simulink model "SiMoDronesBebopRos_student"  (R2021a)
settings: Solver=FixedStepAuto  StartTime=0  StopTime=35  FixedStep=0.005  MaxStep=1e-3  MinStep=5e-5  RelTol=1e-5  AbsTol=1e-5
StopFcn:
  | %data_bebop;
  | save_and_plot_data
values from neighbouring files (symbols this model uses):
  aero =     [test1_p1.mat]    (also in test2_P2.mat; test3_pd.mat; test4_lat.mat; xtest4_lat.mat)
  controlGains =     [test1_p1.mat]    (also in test2_P2.mat; test3_pd.mat; test4_lat.mat; xtest4_lat.mat)
  drone =     [test1_p1.mat]    (also in test2_P2.mat; test3_pd.mat; test4_lat.mat; xtest4_lat.mat)
  init_state =     [test1_p1.mat]    (also in test2_P2.mat; test3_pd.mat; test4_lat.mat; xtest4_lat.mat)
  K = place(A,B,P0)    [Control.m]    (also in test1_p1.mat = [0.637104994903 0.356778797146]; test2_P2.mat = [0.637104994903 0.356778797146]; test3_pd.mat = [0.637104994903 0.356778797146]; test4_lat.mat = [0.637104994903 0.356778797146])
  Kd = 3.806    [Control.m]    (also in test1_p1.mat = 5.726; test2_P2.mat = 5.726; test3_pd.mat = 5.726; test4_lat.mat = 5.726)
  Kdd = 2*sg*om*tau-1    (= 0.98)    [Control.m]    (also in test1_p1.mat = 1.509; test2_P2.mat = 1.509; test3_pd.mat; test4_lat.mat = 1.509)
  Ki = 37.39    [Control.m]    (also in test1_p1.mat = 83.71; test2_P2.mat = 83.71; test3_pd.mat = 83.71; test4_lat.mat = 83.71)
  Kp = 25.23    [Control.m]    (also in test1_p1.mat = 43.79; test2_P2.mat = 43.79; test3_pd.mat = 43.79; test4_lat.mat = 43.79)
  Kp1 = 4    [Control.m]    (also in test1_p1.mat; test2_P2.mat; test3_pd.mat; test4_lat.mat)
  Kp2 = 5.2071    [Control.m]    (also in test1_p1.mat; test2_P2.mat; test3_pd.mat; test4_lat.mat)
  Kpd = tau*om^2    (= 6.0612244898)    [Control.m]    (also in test1_p1.mat = 12.82; test2_P2.mat = 12.82; test3_pd.mat; test4_lat.mat = 12.82)
  measure =     [test1_p1.mat]    (also in test2_P2.mat; test3_pd.mat; test4_lat.mat; xtest4_lat.mat)
  motor =     [test1_p1.mat]    (also in test2_P2.mat; test3_pd.mat; test4_lat.mat; xtest4_lat.mat)
  N = K1    [Control.m]    (also in test1_p1.mat = 0.637104994903; test2_P2.mat = 0.637104994903; test3_pd.mat = 0.637104994903; test4_lat.mat = 0.637104994903)
  tau = 0.33    [Control.m]    (also in test1_p1.mat; test2_P2.mat; test3_pd.mat; test4_lat.mat)
  Te = Ts_optitrack    (= 0.02)    [Startup_bebop_ros.m]    (also in test1_p1.mat; test2_P2.mat; test3_pd.mat; test4_lat.mat)
  Te_topics_empty = 0.1    [Startup_bebop_ros.m]    (also in test1_p1.mat; test2_P2.mat; test3_pd.mat; test4_lat.mat)
  Ts_bebop = 5e-3    (= 0.005)    [Startup_bebop_ros.m]    (also in test1_p1.mat; test2_P2.mat; test3_pd.mat; test4_lat.mat)
  Ts_bebop_feedback = 2e-1    (= 0.2)    [Startup_bebop_ros.m]    (also in test1_p1.mat; test2_P2.mat; test3_pd.mat; test4_lat.mat)
  Ts_optitrack = 2e-2    (= 0.02)    [Startup_bebop_ros.m]    (also in test1_p1.mat; test2_P2.mat; test3_pd.mat; test4_lat.mat)
undefined symbols (not defined in the file or in its folder): Angular, DiscIntNeverNeededParam, gcbh, Linear, sigbuilder_block, sldros_modeswitch
libraries: robotlib x15, simulink x9, pid_lib x8, vrlib x5, lib_isae_drones x4, aerolibanimutils x2, sharedtransform x2, aerolibobsolete x1, drones x1
(part 2 of 3)

== system SiMoDronesBebopRos_student/BEBOP/Model/Model/Bus Mapping1 ==
  Position : Inport
  Velocity : Inport  Port=2
  Attitude : Inport  Port=3
  Omega : Inport  Port=4
  Bus Creator : BusCreator  Inputs=12  OutDataTypeStr=Bus: BUS_bebop_pos_att
  Demux{,1..3} (4 alike) : Demux  Outputs=3
  pos_att_NED : Outport  OutDataTypeStr=Bus: BUS_bebop_pos_att  VectorParamsAs1DForOutWhenUnconnected=off
  wires:
  Position/1 -> Demux/1
  Demux/1 -> Bus Creator/1  "X"
  Demux/3 -> Bus Creator/3  "Z"
  Demux/2 -> Bus Creator/2  "Y"
  Velocity/1 -> Demux1/1
  Demux1/1 -> Bus Creator/4  "VX"
  Demux1/2 -> Bus Creator/5  "VY"
  Demux1/3 -> Bus Creator/6  "VZ"
  Attitude/1 -> Demux2/1
  Demux2/1 -> Bus Creator/7  "Phi"
  Demux2/2 -> Bus Creator/8  "Theta"
  Demux2/3 -> Bus Creator/9  "Psi"
  Omega/1 -> Demux3/1
  Demux3/1 -> Bus Creator/10  "p"
  Demux3/2 -> Bus Creator/11  "q"
  Demux3/3 -> Bus Creator/12  "r"
  Bus Creator/1 -> pos_att_NED/1

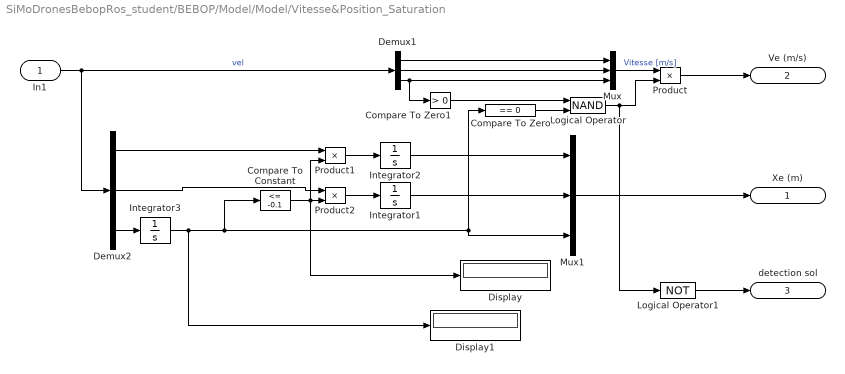
== system SiMoDronesBebopRos_student/BEBOP/Model/Model/Vitesse&Position_Saturation ==
  In1 : Inport
  Compare To Constant : simulink/Logic and Bit Operations/Compare To Constant  relop=<=  const=-0.1  OutDataTypeStr=boolean
  Compare To Zero : simulink/Logic and Bit Operations/Compare To Zero  relop===  OutDataTypeStr=boolean
  Compare To Zero1 : simulink/Logic and Bit Operations/Compare To Zero  relop=>  OutDataTypeStr=boolean
  Demux1 : Demux  Outputs=3
  Demux2 : Demux  Outputs=3
  Display : Display
  Display1 : Display
  Integrator1 : Integrator  InitialCondition=init_state.Pterre0(2)  UpperSaturationLimit=[Inf Inf 0]
  Integrator2 : Integrator  InitialCondition=init_state.Pterre0(1)  UpperSaturationLimit=[Inf Inf 0]
  Integrator3 : Integrator  InitialCondition=init_state.Pterre0(3)  LimitOutput=on  UpperSaturationLimit=[0]
  Logical Operator : Logic  Operator=NAND  AllPortsSameDT=off  OutDataTypeStr=boolean
  Logical Operator1 : Logic  Operator=NOT  AllPortsSameDT=off  OutDataTypeStr=boolean
  Mux : Mux  Inputs=3
  Mux1 : Mux  Inputs=3
  Product : Product  RndMeth=Zero
  Product1 : Product  RndMeth=Zero
  Product2 : Product  RndMeth=Zero
  Xe (m) : Outport  VectorParamsAs1DForOutWhenUnconnected=off
  Ve (m/s) : Outport  Port=2  VectorParamsAs1DForOutWhenUnconnected=off
  detection sol : Outport  Port=3  VectorParamsAs1DForOutWhenUnconnected=off
  wires:
  Compare To Zero1/1 -> Logical Operator/1
  Compare To Zero/1 -> Logical Operator/2
  Demux1/1 -> Mux/1
  Demux1/2 -> Mux/2
  Demux1/3 -> Mux/3, Compare To Zero1/1
  In1/1 -> Demux1/1, Demux2/1  "vel"
  Mux/1 -> Product/1  "Vitesse [m/s]"
  Product/1 -> Ve (m/s)/1
  Integrator1/1 -> Mux1/2
  Demux2/3 -> Integrator3/1
  Integrator3/1 -> Display1/1, Compare To Constant/1, Compare To Zero/1, Mux1/3
  Integrator2/1 -> Mux1/1
  Product1/1 -> Integrator2/1
  Demux2/1 -> Product1/1
  Product2/1 -> Integrator1/1
  Demux2/2 -> Product2/1
  Compare To Constant/1 -> Product1/2, Display/1, Product2/2
  Mux1/1 -> Xe (m)/1
  Logical Operator/1 -> Logical Operator1/1, Product/2
  Logical Operator1/1 -> detection sol/1

== system SiMoDronesBebopRos_student/Guidance & Control /Position Control/Control z/P controller - 1st order system ==
  note: Model
  note: Bebop simulation
  Zref : Inport
  Vz : Inport  Port=2
  Z : Inport  Port=3
  Integrator : Integrator  InitialCondition=-1.5
  PID Controller : pid_lib/PID Controller  Controller=P  Form=Parallel  TimeDomain=Discrete-time  UseExternalTs=off  SampleTime=0.02  IntegratorMethod=Forward Euler  FilterMethod=Forward Euler  ControllerParametersSource=internal  P=Kp1  I=1  D=0.9800  UseFilter=off  N=100  TunerSelectOption=Transfer Function Based (PID Tuner App)  InitialConditionSource=internal  InitialConditionForIntegrator=0  InitialConditionForFilter=0  DifferentiatorICPrevScaledInput=0  ExternalReset=none  TrackingMode=off  Kt=1  LimitOutput=off  SatLimitsSource=internal  UpperSaturationLimit=inf  LowerSaturationLimit=-inf  LinearizeAsGain=on  AntiWindupMode=none  Kb=1  POutMin=[]  POutMax=[]  IOutMin=[]  IOutMax=[]  DOutMin=[]  DOutMax=[]  NOutMin=[]  NOutMax=[]  SumOutMin=[]  SumOutMax=[]  SaturationOutMin=[]  SaturationOutMax=[]  PParamMin=[]  PParamMax=[]  IParamMin=[]  IParamMax=[]  DParamMin=[]  DParamMax=[]  NParamMin=[]  NParamMax=[]  KbParamMin=[]  KbParamMax=[]  KtParamMin=[]  KtParamMax=[]  KbOutMin=[]  KbOutMax=[]  KtOutMin=[]  KtOutMax=[]  IntegratorOutMin=[]  IntegratorOutMax=[]  FilterOutMin=[]  FilterOutMax=[]  SumI1OutMin=[]  SumI1OutMax=[]  SumI2OutMin=[]  SumI2OutMax=[]  SumI3OutMin=[]  SumI3OutMax=[]  SumI4OutMin=[]  SumI4OutMax=[]  SumDOutMin=[]  SumDOutMax=[]  DifferentiatorOutMin=[]  DifferentiatorOutMax=[]  FilterDiffOutCoefMin=[]  FilterDiffOutCoefMax=[]  ReciprocalOutMin=[]  ReciprocalOutMax=[]  SumDenOutMin=[]  SumDenOutMax=[]  SumNumOutMin=[]  SumNumOutMax=[]  DivideOutMin=[]  DivideOutMax=[]  UdiffTsProdOutMin=[]  UdiffTsProdOutMax=[]  NTsProdOutMin=[]  NTsProdOutMax=[]  UintegralTsProdOutMin=[]  UintegralTsProdOutMax=[]  UngainTsProdOutMin=[]  UngainTsProdOutMax=[]  IntegratorContinuousStateAttributes=''  IntegratorStateMustResolveToSignalObject=off  IntegratorRTWStateStorageClass=Auto  FilterContinuousStateAttributes=''  FilterStateMustResolveToSignalObject=off  FilterRTWStateStorageClass=Auto  ParallelPVariant=InternalParameters  IdealPVariant=Disabled  IVariant=Disabled  DVariant=Disabled  IntegratorVariant=Disabled  SatVariant=Disabled  AWVariant=Disabled  PCopyVariant=Disabled  TRVariant=Disabled  FdbkBlocksVariant=Forward  IdealPFdbkVariant=Disabled  SatFdbkVariant=Disabled  DerivativeFilterVariant=Disabled  NVariant=Disabled  NCopyVariant=Disabled_SignalSpec  FilterICVariant=Disabled  IntegratorICVariant=Disabled  ExternalResetVariant=Disabled  TRSumVariant=Passthrough  SumFdbkVariant=Disabled  SumVariant=Passthrough_P  TsampFilterVariant=InternalTs  TsampNgainVariant=Passthrough  TsampIntegralVariant=Disabled_SignalSpec  ExternalSaturationOutDataTypeStr=Inherit: Same as second input
  PID Controller1 : pid_lib/PID Controller  Controller=P  Form=Parallel  TimeDomain=Discrete-time  UseExternalTs=off  SampleTime=0.02  IntegratorMethod=Forward Euler  FilterMethod=Forward Euler  ControllerParametersSource=internal  P=Kp1  I=1  D=0.9800  UseFilter=off  N=100  TunerSelectOption=Transfer Function Based (PID Tuner App)  InitialConditionSource=internal  InitialConditionForIntegrator=0  InitialConditionForFilter=0  DifferentiatorICPrevScaledInput=0  ExternalReset=none  TrackingMode=off  Kt=1  LimitOutput=off  SatLimitsSource=internal  UpperSaturationLimit=inf  LowerSaturationLimit=-inf  LinearizeAsGain=on  AntiWindupMode=none  Kb=1  POutMin=[]  POutMax=[]  IOutMin=[]  IOutMax=[]  DOutMin=[]  DOutMax=[]  NOutMin=[]  NOutMax=[]  SumOutMin=[]  SumOutMax=[]  SaturationOutMin=[]  SaturationOutMax=[]  PParamMin=[]  PParamMax=[]  IParamMin=[]  IParamMax=[]  DParamMin=[]  DParamMax=[]  NParamMin=[]  NParamMax=[]  KbParamMin=[]  KbParamMax=[]  KtParamMin=[]  KtParamMax=[]  KbOutMin=[]  KbOutMax=[]  KtOutMin=[]  KtOutMax=[]  IntegratorOutMin=[]  IntegratorOutMax=[]  FilterOutMin=[]  FilterOutMax=[]  SumI1OutMin=[]  SumI1OutMax=[]  SumI2OutMin=[]  SumI2OutMax=[]  SumI3OutMin=[]  SumI3OutMax=[]  SumI4OutMin=[]  SumI4OutMax=[]  SumDOutMin=[]  SumDOutMax=[]  DifferentiatorOutMin=[]  DifferentiatorOutMax=[]  FilterDiffOutCoefMin=[]  FilterDiffOutCoefMax=[]  ReciprocalOutMin=[]  ReciprocalOutMax=[]  SumDenOutMin=[]  SumDenOutMax=[]  SumNumOutMin=[]  SumNumOutMax=[]  DivideOutMin=[]  DivideOutMax=[]  UdiffTsProdOutMin=[]  UdiffTsProdOutMax=[]  NTsProdOutMin=[]  NTsProdOutMax=[]  UintegralTsProdOutMin=[]  UintegralTsProdOutMax=[]  UngainTsProdOutMin=[]  UngainTsProdOutMax=[]  IntegratorContinuousStateAttributes=''  IntegratorStateMustResolveToSignalObject=off  IntegratorRTWStateStorageClass=Auto  FilterContinuousStateAttributes=''  FilterStateMustResolveToSignalObject=off  FilterRTWStateStorageClass=Auto  ParallelPVariant=InternalParameters  IdealPVariant=Disabled  IVariant=Disabled  DVariant=Disabled  IntegratorVariant=Disabled  SatVariant=Disabled  AWVariant=Disabled  PCopyVariant=Disabled  TRVariant=Disabled  FdbkBlocksVariant=Forward  IdealPFdbkVariant=Disabled  SatFdbkVariant=Disabled  DerivativeFilterVariant=Disabled  NVariant=Disabled  NCopyVariant=Disabled_SignalSpec  FilterICVariant=Disabled  IntegratorICVariant=Disabled  ExternalResetVariant=Disabled  TRSumVariant=Passthrough  SumFdbkVariant=Disabled  SumVariant=Passthrough_P  TsampFilterVariant=InternalTs  TsampNgainVariant=Passthrough  TsampIntegralVariant=Disabled_SignalSpec  ExternalSaturationOutDataTypeStr=Inherit: Same as second input
  Scope : Scope  NumInputPorts=2
  Scope1 : Scope  NumInputPorts=2
  Sum : Sum  Inputs=|+-
  Sum1 : Sum  Inputs=|+-
  To Workspace : ToWorkspace  VariableName=zmodel_P1  SaveFormat=Timeseries  SampleTime=0.02
  VZref : Outport  OutputWhenDisabled=reset  InitialOutput=0  VectorParamsAs1DForOutWhenUnconnected=off
  wires:
  Z/1 -> Sum/2, Scope/1  "zopti"
  PID Controller/1 -> VZref/1
  Sum/1 -> PID Controller/1
  Integrator/1 -> To Workspace/1, Scope/2, Sum1/2  "zmodel"
  PID Controller1/1 -> Scope1/2, Integrator/1  "Vzmodel"
  Vz/1 -> Scope1/1
  Sum1/1 -> PID Controller1/1
  Zref/1 -> Sum1/1, Sum/1

== system SiMoDronesBebopRos_student/Guidance & Control /Position Control/Control z/P controller - 2nd order system ==
  note: Model
  note: Bebop simulation
  Zref : Inport
  Vz : Inport  Port=2
  Z : Inport  Port=3
  Actuator dynamics : TransferFcn  Denominator=[tau 1]
  Integrator : Integrator  InitialCondition=-1.5
  PID Controller : pid_lib/PID Controller  Controller=P  Form=Parallel  TimeDomain=Discrete-time  UseExternalTs=off  SampleTime=0.02  IntegratorMethod=Forward Euler  FilterMethod=Forward Euler  ControllerParametersSource=internal  P=Kp2  I=1  D=1  UseFilter=on  N=100  TunerSelectOption=Transfer Function Based (PID Tuner App)  InitialConditionSource=internal  InitialConditionForIntegrator=0  InitialConditionForFilter=0  DifferentiatorICPrevScaledInput=0  ExternalReset=none  TrackingMode=off  Kt=1  LimitOutput=off  SatLimitsSource=internal  UpperSaturationLimit=inf  LowerSaturationLimit=-inf  LinearizeAsGain=on  AntiWindupMode=none  Kb=1  POutMin=[]  POutMax=[]  IOutMin=[]  IOutMax=[]  DOutMin=[]  DOutMax=[]  NOutMin=[]  NOutMax=[]  SumOutMin=[]  SumOutMax=[]  SaturationOutMin=[]  SaturationOutMax=[]  PParamMin=[]  PParamMax=[]  IParamMin=[]  IParamMax=[]  DParamMin=[]  DParamMax=[]  NParamMin=[]  NParamMax=[]  KbParamMin=[]  KbParamMax=[]  KtParamMin=[]  KtParamMax=[]  KbOutMin=[]  KbOutMax=[]  KtOutMin=[]  KtOutMax=[]  IntegratorOutMin=[]  IntegratorOutMax=[]  FilterOutMin=[]  FilterOutMax=[]  SumI1OutMin=[]  SumI1OutMax=[]  SumI2OutMin=[]  SumI2OutMax=[]  SumI3OutMin=[]  SumI3OutMax=[]  SumI4OutMin=[]  SumI4OutMax=[]  SumDOutMin=[]  SumDOutMax=[]  DifferentiatorOutMin=[]  DifferentiatorOutMax=[]  FilterDiffOutCoefMin=[]  FilterDiffOutCoefMax=[]  ReciprocalOutMin=[]  ReciprocalOutMax=[]  SumDenOutMin=[]  SumDenOutMax=[]  SumNumOutMin=[]  SumNumOutMax=[]  DivideOutMin=[]  DivideOutMax=[]  UdiffTsProdOutMin=[]  UdiffTsProdOutMax=[]  NTsProdOutMin=[]  NTsProdOutMax=[]  UintegralTsProdOutMin=[]  UintegralTsProdOutMax=[]  UngainTsProdOutMin=[]  UngainTsProdOutMax=[]  IntegratorContinuousStateAttributes=''  IntegratorStateMustResolveToSignalObject=off  IntegratorRTWStateStorageClass=Auto  FilterContinuousStateAttributes=''  FilterStateMustResolveToSignalObject=off  FilterRTWStateStorageClass=Auto  ParallelPVariant=InternalParameters  IdealPVariant=Disabled  IVariant=Disabled  DVariant=Disabled  IntegratorVariant=Disabled  SatVariant=Disabled  AWVariant=Disabled  PCopyVariant=Disabled  TRVariant=Disabled  FdbkBlocksVariant=Forward  IdealPFdbkVariant=Disabled  SatFdbkVariant=Disabled  DerivativeFilterVariant=Disabled  NVariant=Disabled  NCopyVariant=Disabled_SignalSpec  FilterICVariant=Disabled  IntegratorICVariant=Disabled  ExternalResetVariant=Disabled  TRSumVariant=Passthrough  SumFdbkVariant=Disabled  SumVariant=Passthrough_P  TsampFilterVariant=InternalTs  TsampNgainVariant=Passthrough  TsampIntegralVariant=Disabled_SignalSpec  ExternalSaturationOutDataTypeStr=Inherit: Same as second input
  PID Controller1 : pid_lib/PID Controller  Controller=P  Form=Parallel  TimeDomain=Discrete-time  UseExternalTs=off  SampleTime=0.02  IntegratorMethod=Forward Euler  FilterMethod=Forward Euler  ControllerParametersSource=internal  P=Kp2  I=1  D=1  UseFilter=on  N=100  TunerSelectOption=Transfer Function Based (PID Tuner App)  InitialConditionSource=internal  InitialConditionForIntegrator=0  InitialConditionForFilter=0  DifferentiatorICPrevScaledInput=0  ExternalReset=none  TrackingMode=off  Kt=1  LimitOutput=off  SatLimitsSource=internal  UpperSaturationLimit=inf  LowerSaturationLimit=-inf  LinearizeAsGain=on  AntiWindupMode=none  Kb=1  POutMin=[]  POutMax=[]  IOutMin=[]  IOutMax=[]  DOutMin=[]  DOutMax=[]  NOutMin=[]  NOutMax=[]  SumOutMin=[]  SumOutMax=[]  SaturationOutMin=[]  SaturationOutMax=[]  PParamMin=[]  PParamMax=[]  IParamMin=[]  IParamMax=[]  DParamMin=[]  DParamMax=[]  NParamMin=[]  NParamMax=[]  KbParamMin=[]  KbParamMax=[]  KtParamMin=[]  KtParamMax=[]  KbOutMin=[]  KbOutMax=[]  KtOutMin=[]  KtOutMax=[]  IntegratorOutMin=[]  IntegratorOutMax=[]  FilterOutMin=[]  FilterOutMax=[]  SumI1OutMin=[]  SumI1OutMax=[]  SumI2OutMin=[]  SumI2OutMax=[]  SumI3OutMin=[]  SumI3OutMax=[]  SumI4OutMin=[]  SumI4OutMax=[]  SumDOutMin=[]  SumDOutMax=[]  DifferentiatorOutMin=[]  DifferentiatorOutMax=[]  FilterDiffOutCoefMin=[]  FilterDiffOutCoefMax=[]  ReciprocalOutMin=[]  ReciprocalOutMax=[]  SumDenOutMin=[]  SumDenOutMax=[]  SumNumOutMin=[]  SumNumOutMax=[]  DivideOutMin=[]  DivideOutMax=[]  UdiffTsProdOutMin=[]  UdiffTsProdOutMax=[]  NTsProdOutMin=[]  NTsProdOutMax=[]  UintegralTsProdOutMin=[]  UintegralTsProdOutMax=[]  UngainTsProdOutMin=[]  UngainTsProdOutMax=[]  IntegratorContinuousStateAttributes=''  IntegratorStateMustResolveToSignalObject=off  IntegratorRTWStateStorageClass=Auto  FilterContinuousStateAttributes=''  FilterStateMustResolveToSignalObject=off  FilterRTWStateStorageClass=Auto  ParallelPVariant=InternalParameters  IdealPVariant=Disabled  IVariant=Disabled  DVariant=Disabled  IntegratorVariant=Disabled  SatVariant=Disabled  AWVariant=Disabled  PCopyVariant=Disabled  TRVariant=Disabled  FdbkBlocksVariant=Forward  IdealPFdbkVariant=Disabled  SatFdbkVariant=Disabled  DerivativeFilterVariant=Disabled  NVariant=Disabled  NCopyVariant=Disabled_SignalSpec  FilterICVariant=Disabled  IntegratorICVariant=Disabled  ExternalResetVariant=Disabled  TRSumVariant=Passthrough  SumFdbkVariant=Disabled  SumVariant=Passthrough_P  TsampFilterVariant=InternalTs  TsampNgainVariant=Passthrough  TsampIntegralVariant=Disabled_SignalSpec  ExternalSaturationOutDataTypeStr=Inherit: Same as second input
  Scope : Scope  NumInputPorts=2
  Scope1 : Scope  NumInputPorts=2
  Sum : Sum  Inputs=|+-
  Sum1 : Sum  Inputs=|+-
  To Workspace : ToWorkspace  VariableName=zmodel_P2  SaveFormat=Timeseries  SampleTime=0.02
  VZref : Outport  OutputWhenDisabled=reset  InitialOutput=0  VectorParamsAs1DForOutWhenUnconnected=off
  wires:
  Z/1 -> Sum/2, Scope/1  "zopti"
  Zref/1 -> Sum1/1, Sum/1
  PID Controller/1 -> VZref/1
  Sum/1 -> PID Controller/1
  Integrator/1 -> Sum1/2, To Workspace/1, Scope/2  "zmodel"
  Vz/1 -> Scope1/1
  Sum1/1 -> PID Controller1/1
  PID Controller1/1 -> Actuator dynamics/1  "Vzmodel"
  Actuator dynamics/1 -> Scope1/2, Integrator/1

== system SiMoDronesBebopRos_student/Guidance & Control /Position Control/Control z/PD controller - 2nd order system ==
  note: Model
  note: Bebop simulation
  Zref : Inport
  Vz : Inport  Port=2
  Z : Inport  Port=3
  Actuator dynamics : TransferFcn  Denominator=[tau 1]
  Integrator : Integrator  InitialCondition=-1.5
  PID Controller : pid_lib/PID Controller  Controller=PD  Form=Parallel  TimeDomain=Discrete-time  UseExternalTs=off  SampleTime=0.02  IntegratorMethod=Forward Euler  FilterMethod=Forward Euler  ControllerParametersSource=internal  P=Kpd  I=1  D=Kdd  UseFilter=off  N=100  TunerSelectOption=Transfer Function Based (PID Tuner App)  InitialConditionSource=internal  InitialConditionForIntegrator=0  InitialConditionForFilter=0  DifferentiatorICPrevScaledInput=0  ExternalReset=none  TrackingMode=off  Kt=1  LimitOutput=off  SatLimitsSource=internal  UpperSaturationLimit=inf  LowerSaturationLimit=-inf  LinearizeAsGain=on  AntiWindupMode=none  Kb=1  POutMin=[]  POutMax=[]  IOutMin=[]  IOutMax=[]  DOutMin=[]  DOutMax=[]  NOutMin=[]  NOutMax=[]  SumOutMin=[]  SumOutMax=[]  SaturationOutMin=[]  SaturationOutMax=[]  PParamMin=[]  PParamMax=[]  IParamMin=[]  IParamMax=[]  DParamMin=[]  DParamMax=[]  NParamMin=[]  NParamMax=[]  KbParamMin=[]  KbParamMax=[]  KtParamMin=[]  KtParamMax=[]  KbOutMin=[]  KbOutMax=[]  KtOutMin=[]  KtOutMax=[]  IntegratorOutMin=[]  IntegratorOutMax=[]  FilterOutMin=[]  FilterOutMax=[]  SumI1OutMin=[]  SumI1OutMax=[]  SumI2OutMin=[]  SumI2OutMax=[]  SumI3OutMin=[]  SumI3OutMax=[]  SumI4OutMin=[]  SumI4OutMax=[]  SumDOutMin=[]  SumDOutMax=[]  DifferentiatorOutMin=[]  DifferentiatorOutMax=[]  FilterDiffOutCoefMin=[]  FilterDiffOutCoefMax=[]  ReciprocalOutMin=[]  ReciprocalOutMax=[]  SumDenOutMin=[]  SumDenOutMax=[]  SumNumOutMin=[]  SumNumOutMax=[]  DivideOutMin=[]  DivideOutMax=[]  UdiffTsProdOutMin=[]  UdiffTsProdOutMax=[]  NTsProdOutMin=[]  NTsProdOutMax=[]  UintegralTsProdOutMin=[]  UintegralTsProdOutMax=[]  UngainTsProdOutMin=[]  UngainTsProdOutMax=[]  IntegratorContinuousStateAttributes=''  IntegratorStateMustResolveToSignalObject=off  IntegratorRTWStateStorageClass=Auto  FilterContinuousStateAttributes=''  FilterStateMustResolveToSignalObject=off  FilterRTWStateStorageClass=Auto  ParallelPVariant=InternalParameters  IdealPVariant=Disabled  IVariant=Disabled  DVariant=InternalParameters  IntegratorVariant=Disabled  SatVariant=Disabled  AWVariant=Disabled  PCopyVariant=Disabled  TRVariant=Disabled  FdbkBlocksVariant=Forward  IdealPFdbkVariant=Disabled  SatFdbkVariant=Disabled  DerivativeFilterVariant=Differentiator  NVariant=Passthrough  NCopyVariant=Disabled_SignalSpec  FilterICVariant=InternalICsDifferentiator  IntegratorICVariant=Disabled  ExternalResetVariant=Disabled  TRSumVariant=Passthrough  SumFdbkVariant=Disabled  SumVariant=Sum_PD  TsampFilterVariant=InternalTs  TsampNgainVariant=Passthrough  TsampIntegralVariant=Disabled_SignalSpec  ExternalSaturationOutDataTypeStr=Inherit: Same as second input
  PID Controller1 : pid_lib/PID Controller  Controller=PD  Form=Parallel  TimeDomain=Discrete-time  UseExternalTs=off  SampleTime=0.02  IntegratorMethod=Forward Euler  FilterMethod=Forward Euler  ControllerParametersSource=internal  P=Kpd  I=1  D=Kdd  UseFilter=off  N=100  TunerSelectOption=Transfer Function Based (PID Tuner App)  InitialConditionSource=internal  InitialConditionForIntegrator=0  InitialConditionForFilter=0  DifferentiatorICPrevScaledInput=0  ExternalReset=none  TrackingMode=off  Kt=1  LimitOutput=off  SatLimitsSource=internal  UpperSaturationLimit=inf  LowerSaturationLimit=-inf  LinearizeAsGain=on  AntiWindupMode=none  Kb=1  POutMin=[]  POutMax=[]  IOutMin=[]  IOutMax=[]  DOutMin=[]  DOutMax=[]  NOutMin=[]  NOutMax=[]  SumOutMin=[]  SumOutMax=[]  SaturationOutMin=[]  SaturationOutMax=[]  PParamMin=[]  PParamMax=[]  IParamMin=[]  IParamMax=[]  DParamMin=[]  DParamMax=[]  NParamMin=[]  NParamMax=[]  KbParamMin=[]  KbParamMax=[]  KtParamMin=[]  KtParamMax=[]  KbOutMin=[]  KbOutMax=[]  KtOutMin=[]  KtOutMax=[]  IntegratorOutMin=[]  IntegratorOutMax=[]  FilterOutMin=[]  FilterOutMax=[]  SumI1OutMin=[]  SumI1OutMax=[]  SumI2OutMin=[]  SumI2OutMax=[]  SumI3OutMin=[]  SumI3OutMax=[]  SumI4OutMin=[]  SumI4OutMax=[]  SumDOutMin=[]  SumDOutMax=[]  DifferentiatorOutMin=[]  DifferentiatorOutMax=[]  FilterDiffOutCoefMin=[]  FilterDiffOutCoefMax=[]  ReciprocalOutMin=[]  ReciprocalOutMax=[]  SumDenOutMin=[]  SumDenOutMax=[]  SumNumOutMin=[]  SumNumOutMax=[]  DivideOutMin=[]  DivideOutMax=[]  UdiffTsProdOutMin=[]  UdiffTsProdOutMax=[]  NTsProdOutMin=[]  NTsProdOutMax=[]  UintegralTsProdOutMin=[]  UintegralTsProdOutMax=[]  UngainTsProdOutMin=[]  UngainTsProdOutMax=[]  IntegratorContinuousStateAttributes=''  IntegratorStateMustResolveToSignalObject=off  IntegratorRTWStateStorageClass=Auto  FilterContinuousStateAttributes=''  FilterStateMustResolveToSignalObject=off  FilterRTWStateStorageClass=Auto  ParallelPVariant=InternalParameters  IdealPVariant=Disabled  IVariant=Disabled  DVariant=InternalParameters  IntegratorVariant=Disabled  SatVariant=Disabled  AWVariant=Disabled  PCopyVariant=Disabled  TRVariant=Disabled  FdbkBlocksVariant=Forward  IdealPFdbkVariant=Disabled  SatFdbkVariant=Disabled  DerivativeFilterVariant=Differentiator  NVariant=Passthrough  NCopyVariant=Disabled_SignalSpec  FilterICVariant=InternalICsDifferentiator  IntegratorICVariant=Disabled  ExternalResetVariant=Disabled  TRSumVariant=Passthrough  SumFdbkVariant=Disabled  SumVariant=Sum_PD  TsampFilterVariant=InternalTs  TsampNgainVariant=Passthrough  TsampIntegralVariant=Disabled_SignalSpec  ExternalSaturationOutDataTypeStr=Inherit: Same as second input
  Scope : Scope  NumInputPorts=2
  Scope1 : Scope  NumInputPorts=2
  Sum : Sum  Inputs=|+-
  Sum1 : Sum  Inputs=|+-
  To Workspace : ToWorkspace  VariableName=zmodel_PD2  SaveFormat=Timeseries  SampleTime=0.02
  VZref : Outport  OutputWhenDisabled=reset  InitialOutput=0  VectorParamsAs1DForOutWhenUnconnected=off
  wires:
  Z/1 -> Sum/2, Scope/1  "zopti"
  Zref/1 -> Sum1/1, Sum/1
  PID Controller/1 -> VZref/1
  Sum/1 -> PID Controller/1
  Integrator/1 -> Sum1/2, To Workspace/1, Scope/2  "zmodel"
  Vz/1 -> Scope1/1
  Sum1/1 -> PID Controller1/1
  PID Controller1/1 -> Actuator dynamics/1  "Vzmodel"
  Actuator dynamics/1 -> Scope1/2, Integrator/1

== system SiMoDronesBebopRos_student/Guidance & Control /Position Control/Control z/PID controller - 2nd order system ==
  note: Model
  note: Bebop simulation
  Zref : Inport
  Vz : Inport  Port=2
  Z : Inport  Port=3
  Actuator dynamics : TransferFcn  Denominator=[tau 1]
  Integrator : Integrator  InitialCondition=-1.5
  PID Controller2 : pid_lib/PID Controller  Controller=PID  Form=Parallel  TimeDomain=Discrete-time  UseExternalTs=off  SampleTime=0.02  IntegratorMethod=Forward Euler  FilterMethod=Forward Euler  ControllerParametersSource=internal  P=Kp  I=Ki  D=Kd  UseFilter=off  N=79.7925316192384  TunerSelectOption=Transfer Function Based (PID Tuner App)  InitialConditionSource=internal  InitialConditionForIntegrator=0  InitialConditionForFilter=0  DifferentiatorICPrevScaledInput=0  ExternalReset=none  TrackingMode=off  Kt=1  LimitOutput=off  SatLimitsSource=internal  UpperSaturationLimit=inf  LowerSaturationLimit=-inf  LinearizeAsGain=on  AntiWindupMode=none  Kb=1  POutMin=[]  POutMax=[]  IOutMin=[]  IOutMax=[]  DOutMin=[]  DOutMax=[]  NOutMin=[]  NOutMax=[]  SumOutMin=[]  SumOutMax=[]  SaturationOutMin=[]  SaturationOutMax=[]  PParamMin=[]  PParamMax=[]  IParamMin=[]  IParamMax=[]  DParamMin=[]  DParamMax=[]  NParamMin=[]  NParamMax=[]  KbParamMin=[]  KbParamMax=[]  KtParamMin=[]  KtParamMax=[]  KbOutMin=[]  KbOutMax=[]  KtOutMin=[]  KtOutMax=[]  IntegratorOutMin=[]  IntegratorOutMax=[]  FilterOutMin=[]  FilterOutMax=[]  SumI1OutMin=[]  SumI1OutMax=[]  SumI2OutMin=[]  SumI2OutMax=[]  SumI3OutMin=[]  SumI3OutMax=[]  SumI4OutMin=[]  SumI4OutMax=[]  SumDOutMin=[]  SumDOutMax=[]  DifferentiatorOutMin=[]  DifferentiatorOutMax=[]  FilterDiffOutCoefMin=[]  FilterDiffOutCoefMax=[]  ReciprocalOutMin=[]  ReciprocalOutMax=[]  SumDenOutMin=[]  SumDenOutMax=[]  SumNumOutMin=[]  SumNumOutMax=[]  DivideOutMin=[]  DivideOutMax=[]  UdiffTsProdOutMin=[]  UdiffTsProdOutMax=[]  NTsProdOutMin=[]  NTsProdOutMax=[]  UintegralTsProdOutMin=[]  UintegralTsProdOutMax=[]  UngainTsProdOutMin=[]  UngainTsProdOutMax=[]  IntegratorContinuousStateAttributes=''  IntegratorStateMustResolveToSignalObject=off  IntegratorRTWStateStorageClass=Auto  FilterContinuousStateAttributes=''  FilterStateMustResolveToSignalObject=off  FilterRTWStateStorageClass=Auto  ParallelPVariant=InternalParameters  IdealPVariant=Disabled  IVariant=InternalParameters  DVariant=InternalParameters  IntegratorVariant=Discrete  SatVariant=Disabled  AWVariant=Passthrough  PCopyVariant=Disabled  TRVariant=Disabled  FdbkBlocksVariant=Forward  IdealPFdbkVariant=Disabled  SatFdbkVariant=Disabled  DerivativeFilterVariant=Differentiator  NVariant=Passthrough  NCopyVariant=Disabled_SignalSpec  FilterICVariant=InternalICsDifferentiator  IntegratorICVariant=InternalICs  ExternalResetVariant=Disabled  TRSumVariant=Passthrough  SumFdbkVariant=Disabled  SumVariant=Sum_PID  TsampFilterVariant=InternalTs  TsampNgainVariant=Passthrough  TsampIntegralVariant=Passthrough  ExternalSaturationOutDataTypeStr=Inherit: Same as second input
  PID Controller3 : pid_lib/PID Controller  Controller=PID  Form=Parallel  TimeDomain=Discrete-time  UseExternalTs=off  SampleTime=0.02  IntegratorMethod=Forward Euler  FilterMethod=Forward Euler  ControllerParametersSource=internal  P=Kp  I=Ki  D=Kd  UseFilter=off  N=79.7925316192384  TunerSelectOption=Transfer Function Based (PID Tuner App)  InitialConditionSource=internal  InitialConditionForIntegrator=0  InitialConditionForFilter=0  DifferentiatorICPrevScaledInput=0  ExternalReset=none  TrackingMode=off  Kt=1  LimitOutput=off  SatLimitsSource=internal  UpperSaturationLimit=inf  LowerSaturationLimit=-inf  LinearizeAsGain=on  AntiWindupMode=none  Kb=1  POutMin=[]  POutMax=[]  IOutMin=[]  IOutMax=[]  DOutMin=[]  DOutMax=[]  NOutMin=[]  NOutMax=[]  SumOutMin=[]  SumOutMax=[]  SaturationOutMin=[]  SaturationOutMax=[]  PParamMin=[]  PParamMax=[]  IParamMin=[]  IParamMax=[]  DParamMin=[]  DParamMax=[]  NParamMin=[]  NParamMax=[]  KbParamMin=[]  KbParamMax=[]  KtParamMin=[]  KtParamMax=[]  KbOutMin=[]  KbOutMax=[]  KtOutMin=[]  KtOutMax=[]  IntegratorOutMin=[]  IntegratorOutMax=[]  FilterOutMin=[]  FilterOutMax=[]  SumI1OutMin=[]  SumI1OutMax=[]  SumI2OutMin=[]  SumI2OutMax=[]  SumI3OutMin=[]  SumI3OutMax=[]  SumI4OutMin=[]  SumI4OutMax=[]  SumDOutMin=[]  SumDOutMax=[]  DifferentiatorOutMin=[]  DifferentiatorOutMax=[]  FilterDiffOutCoefMin=[]  FilterDiffOutCoefMax=[]  ReciprocalOutMin=[]  ReciprocalOutMax=[]  SumDenOutMin=[]  SumDenOutMax=[]  SumNumOutMin=[]  SumNumOutMax=[]  DivideOutMin=[]  DivideOutMax=[]  UdiffTsProdOutMin=[]  UdiffTsProdOutMax=[]  NTsProdOutMin=[]  NTsProdOutMax=[]  UintegralTsProdOutMin=[]  UintegralTsProdOutMax=[]  UngainTsProdOutMin=[]  UngainTsProdOutMax=[]  IntegratorContinuousStateAttributes=''  IntegratorStateMustResolveToSignalObject=off  IntegratorRTWStateStorageClass=Auto  FilterContinuousStateAttributes=''  FilterStateMustResolveToSignalObject=off  FilterRTWStateStorageClass=Auto  ParallelPVariant=InternalParameters  IdealPVariant=Disabled  IVariant=InternalParameters  DVariant=InternalParameters  IntegratorVariant=Discrete  SatVariant=Disabled  AWVariant=Passthrough  PCopyVariant=Disabled  TRVariant=Disabled  FdbkBlocksVariant=Forward  IdealPFdbkVariant=Disabled  SatFdbkVariant=Disabled  DerivativeFilterVariant=Differentiator  NVariant=Passthrough  NCopyVariant=Disabled_SignalSpec  FilterICVariant=InternalICsDifferentiator  IntegratorICVariant=InternalICs  ExternalResetVariant=Disabled  TRSumVariant=Passthrough  SumFdbkVariant=Disabled  SumVariant=Sum_PID  TsampFilterVariant=InternalTs  TsampNgainVariant=Passthrough  TsampIntegralVariant=Passthrough  ExternalSaturationOutDataTypeStr=Inherit: Same as second input
  Scope : Scope  NumInputPorts=2
  Scope1 : Scope  NumInputPorts=2
  Sum : Sum  Inputs=|+-
  Sum1 : Sum  Inputs=|+-
  To Workspace : ToWorkspace  VariableName=zmodel_PID2  SaveFormat=Timeseries  SampleTime=0.02
  VZref : Outport  OutputWhenDisabled=reset  InitialOutput=0  VectorParamsAs1DForOutWhenUnconnected=off
  wires:
  Z/1 -> Sum/2, Scope/1  "zopti"
  Zref/1 -> Sum1/1, Sum/1
  Sum/1 -> PID Controller3/1
  Integrator/1 -> To Workspace/1, Scope/2, Sum1/2  "zmodel"
  Vz/1 -> Scope1/1
  Sum1/1 -> PID Controller2/1  "Vzmodel"
  Actuator dynamics/1 -> Scope1/2, Integrator/1
  PID Controller2/1 -> Actuator dynamics/1
  PID Controller3/1 -> VZref/1

== system SiMoDronesBebopRos_student/OPTITRACK/Measure /optitrack_/1er ordre ==
  x : Inport
  Gain1 : Gain  Gain=1/tr5
  Gain2 : Gain  Gain=K
  Integrator : Integrator  InitialCondition=init_inte
  Sum4 : Sum  Inputs=|+-
  x_retard : Outport  VectorParamsAs1DForOutWhenUnconnected=off
  wires:
  Gain1/1 -> Integrator/1
  Integrator/1 -> Gain2/1, Sum4/2
  Sum4/1 -> Gain1/1
  x/1 -> Sum4/1
  Gain2/1 -> x_retard/1

== system SiMoDronesBebopRos_student/OPTITRACK/Measure /optitrack_/1er ordre1 ==
  y : Inport
  Gain1 : Gain  Gain=1/tr5
  Gain2 : Gain  Gain=K
  Integrator : Integrator  InitialCondition=init_inte
  Sum4 : Sum  Inputs=|+-
  y_retard : Outport  VectorParamsAs1DForOutWhenUnconnected=off
  wires:
  Gain2/1 -> y_retard/1
  y/1 -> Sum4/1
  Sum4/1 -> Gain1/1
  Integrator/1 -> Sum4/2, Gain2/1
  Gain1/1 -> Integrator/1

== system SiMoDronesBebopRos_student/OPTITRACK/Measure /optitrack_/1er ordre2 ==
  z : Inport
  Gain1 : Gain  Gain=1/tr5
  Gain2 : Gain  Gain=K
  Integrator : Integrator  InitialCondition=init_inte
  Sum4 : Sum  Inputs=|+-
  z_retard : Outport  VectorParamsAs1DForOutWhenUnconnected=off
  wires:
  Gain1/1 -> Integrator/1
  Integrator/1 -> Gain2/1, Sum4/2
  Sum4/1 -> Gain1/1
  z/1 -> Sum4/1
  Gain2/1 -> z_retard/1

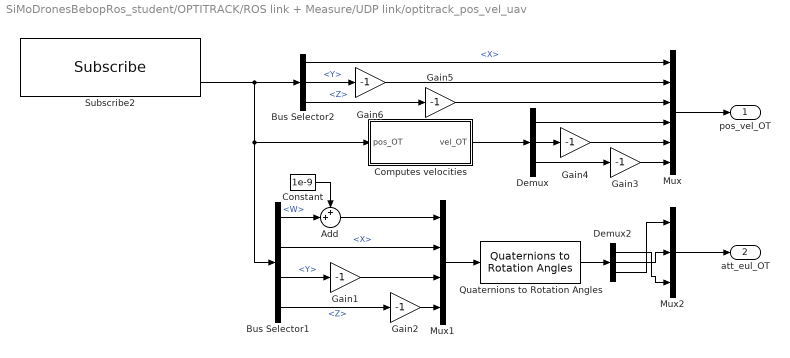
== system SiMoDronesBebopRos_student/OPTITRACK/ROS link + Measure/UDP link/optitrack_pos_vel_uav ==
  Add : Sum  Inputs=++|
  Bus Selector1 : BusSelector  OutputSignals=Pose.Orientation.W,Pose.Orientation.X,Pose.Orientation.Y,Pose.Orientation.Z
  Bus Selector2 : BusSelector  OutputSignals=Pose.Position.X,Pose.Position.Y,Pose.Position.Z
  Computes velocities : Subsystem  TreatAsAtomicUnit=on
  Constant : Constant  Value=1e-9  SampleTime=-1
  Demux : Demux  Outputs=3
  Demux2 : Demux  Outputs=3
  Gain{1..6} (6 alike) : Gain  Gain=-1
  Mux : Mux  Inputs=6
  Mux1 : Mux
  Mux2 : Mux  Inputs=3
  Quaternions to Rotation Angles : sharedtransform/Quaternions to Rotation Angles  rotationOrder=ZYX  aMode=aMode
      settings: SourceProductBaseCode=AE,PW,DR,MT,UV,VE
  Subscribe2 : robotlib/Subscribe  topicSource=Select from ROS network  topic=/bebop/pose  messageType=geometry_msgs/PoseStamped  SampleTime=Te  legacyBusStruct=off  messageQueueLength=1
  pos_vel_OT : Outport  VectorParamsAs1DForOutWhenUnconnected=off
  att_eul_OT : Outport  Port=2  VectorParamsAs1DForOutWhenUnconnected=off
  wires:
  Gain6/1 -> Mux/2
  Gain5/1 -> Mux/3
  Gain4/1 -> Mux/5
  Gain3/1 -> Mux/6
  Gain2/1 -> Mux1/4
  Gain1/1 -> Mux1/3
  Mux/1 -> pos_vel_OT/1
  Bus Selector2/1 -> Mux/1  "<X>"
  Bus Selector2/2 -> Gain6/1  "<Y>"
  Bus Selector2/3 -> Gain5/1  "<Z>"
  Computes velocities/1(vel_OT) -> Demux/1
  Demux/1 -> Mux/4
  Demux/2 -> Gain4/1
  Demux/3 -> Gain3/1
  Mux1/1 -> Quaternions to Rotation Angles/1
  Demux2/2 -> Mux2/2
  Demux2/1 -> Mux2/3
  Demux2/3 -> Mux2/1
  Quaternions to Rotation Angles/1 -> Demux2/1
  Mux2/1 -> att_eul_OT/1
  Bus Selector1/3 -> Gain1/1  "<Y>"
  Bus Selector1/2 -> Mux1/2  "<X>"
  Bus Selector1/4 -> Gain2/1  "<Z>"
  Bus Selector1/1 -> Add/2  "<W>"
  Constant/1 -> Add/1
  Add/1 -> Mux1/1
  Subscribe2/2 -> Bus Selector1/1, Computes velocities/1(pos_OT), Bus Selector2/1

== system SiMoDronesBebopRos_student/BEBOP/Bebop Control/Inner Loop (Parrot)/Bebop onboard control/Régulations ==
  Phi_c : Inport
  Theta_c : Inport  Port=2
  Cde_Lacet : Inport  Port=3
  bebop_sensors : Inport  Port=4  OutDataTypeStr=Bus: BUS_bebop_sensors
  Attitude : Subsystem
  Bus Selector2 : BusSelector  OutputSignals=pitch,roll,q,p,r
  Gain : Gain  Gain=0.001
  Gain1 : Gain  Gain=0.001
  Gain2 : Gain
  Mux : Mux  Inputs=2
  Mux1 : Mux  Inputs=2
  Mux3 : Mux  Inputs=2
  Saturation : Saturate  UpperLimit=controlGains.psi.ratemax  LowerLimit=-controlGains.psi.ratemax
  Sum : Sum  Inputs=|+-
  Out2 : Outport  VectorParamsAs1DForOutWhenUnconnected=off
  Out1 : Outport  Port=2  VectorParamsAs1DForOutWhenUnconnected=off
  Cde_R : Outport  Port=3  VectorParamsAs1DForOutWhenUnconnected=off
  wires:
  Sum/1 -> Gain2/1  "Cde_R"
  Bus Selector2/2 -> Mux/2  "<roll>"
  Phi_c/1 -> Mux1/2  "Phi_c"
  Theta_c/1 -> Mux1/1  "Theta_c"
  Cde_Lacet/1 -> Saturation/1  "Cde_Lacet"
  Bus Selector2/1 -> Mux/1  "<pitch>"
  Mux3/1 -> Attitude/3(rate)
  Mux1/1 -> Attitude/1(refAttitude)
  Mux/1 -> Attitude/2(att_estim)
  Attitude/1(tau_pitch) -> Gain/1
  Attitude/2(tau_roll) -> Gain1/1
  Bus Selector2/3 -> Mux3/1  "<q>"
  Bus Selector2/4 -> Mux3/2  "<p>"
  Gain/1 -> Out1/1  "pitch"
  Gain1/1 -> Out2/1  "roll"
  Saturation/1 -> Sum/1
  Gain2/1 -> Cde_R/1  "yaw"
  bebop_sensors/1 -> Bus Selector2/1
  Bus Selector2/5 -> Sum/2  "<r>"

== system SiMoDronesBebopRos_student/BEBOP/Bebop Control/Inner Loop (Parrot)/Bebop onboard control/Vz control ==
  Vz_d : Inport
  bebop_sensor : Inport  Port=2  OutDataTypeStr=Bus: BUS_bebop_sensors
  bebop_state : Inport  Port=3
  Altitude control : Subsystem
  Bus Selector : BusSelector  OutputSignals=altitude,optical_flow_Vz,pitch,roll
  Discrete Derivative : simulink/Discrete/Discrete Derivative  Commented=on  gainval=1.0  ICPrevScaledInput=0.0  OutMin=[]  OutMax=[]  OutDataType=fixdt(1, 16)  OutScaling=2^-10  DoSatur=off
  Normalized thrust calculation : Subsystem
  Subsystem : Subsystem
  thrust : Outport  VectorParamsAs1DForOutWhenUnconnected=off
  wires:
  Vz_d/1 -> Subsystem/1(Vz_ref)
  Altitude control/1(Vertical thrust (N)) -> Normalized thrust calculation/1(Vertical thrust)
  Normalized thrust calculation/1(Normalized thrust) -> thrust/1
  Subsystem/1(Vz_ref_out) -> Altitude control/1(Vz_ref)
  Subsystem/2(Motor_On) -> Altitude control/2(Motor_On)
  bebop_sensor/1 -> Bus Selector/1
  Bus Selector/2 -> Altitude control/3(Vz_est)  "<optical_flow_Vz>"
  Bus Selector/3 -> Normalized thrust calculation/2(theta)  "<pitch>"
  Bus Selector/4 -> Normalized thrust calculation/3(phi)  "<roll>"
  bebop_state/1 -> Subsystem/2(bebop_state)
  Bus Selector/1 -> Subsystem/3(altitude)  "<altitude>"

== system SiMoDronesBebopRos_student/BEBOP/Bebop Control/Udp send/Topics/Land topic ==
  Enable : EnablePort
  Blank Message : robotlib/Blank Message  messageClass=Message  entityType=std_msgs/Empty  messageType=std_msgs/Empty  SampleTime=Te_topics_empty  legacyBusStruct=off
  Publish : robotlib/Publish  topicSource=Select from ROS network  topic=/bebop/land  messageType=std_msgs/Empty  legacyBusStruct=off  messageQueueLength=1
  wires:
  Blank Message/1 -> Publish/1

== system SiMoDronesBebopRos_student/BEBOP/Bebop Control/Udp send/Topics/takeoff topic ==
  Enable : EnablePort
  Blank Message : robotlib/Blank Message  messageClass=Message  entityType=std_msgs/Empty  messageType=std_msgs/Empty  SampleTime=Te_topics_empty  legacyBusStruct=off
  Publish1 : robotlib/Publish  topicSource=Select from ROS network  topic=/bebop/takeoff  messageType=std_msgs/Empty  legacyBusStruct=off  messageQueueLength=1
  wires:
  Blank Message/1 -> Publish1/1

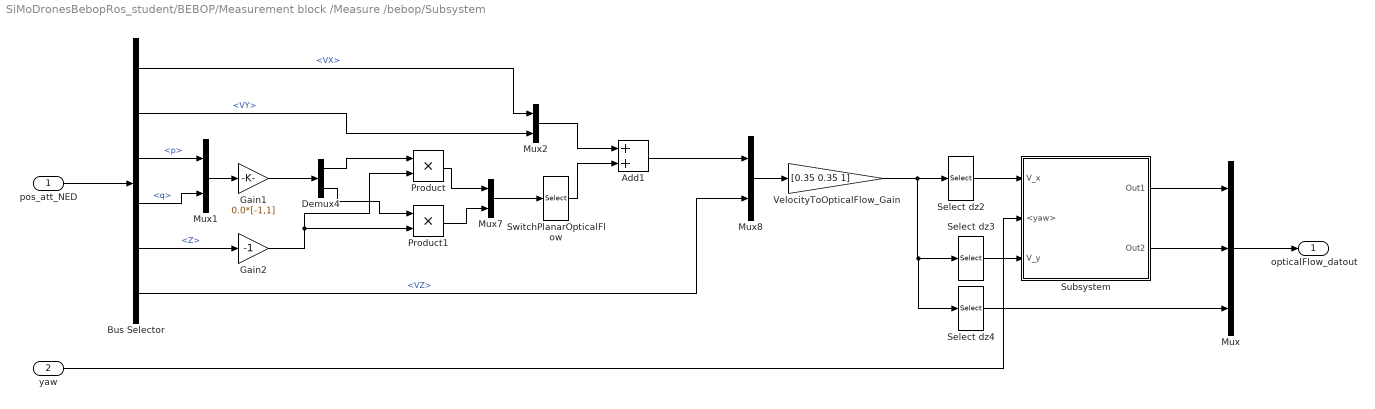
== system SiMoDronesBebopRos_student/BEBOP/Measurement block /Measure /bebop/Subsystem ==
  pos_att_NED : Inport  OutDataTypeStr=Bus: BUS_bebop_pos_att
  yaw : Inport  Port=2
  Add1 : Sum
  Bus Selector : BusSelector  OutputSignals=VX,VY,p,q,Z,VZ
  Demux4 : Demux  Outputs=2
  Gain1 : Gain  Gain=0.0*[-1,1]
  Gain2 : Gain  Gain=-1
  Mux : Mux  Inputs=3
  Mux{1..2,7..8} (4 alike) : Mux  Inputs=2
  Product : Product
  Product1 : Product
  Select dz2 : Selector  InputPortWidth=3  IndexOptions=Index vector (dialog)  Indices=1  OutputSizes=1
  Select dz3 : Selector  InputPortWidth=3  IndexOptions=Index vector (dialog)  Indices=2  OutputSizes=1
  Select dz4 : Selector  InputPortWidth=3  IndexOptions=Index vector (dialog)  Indices=3  OutputSizes=1
  Subsystem : Subsystem
  SwitchPlanarOpticalFlow : Selector  InputPortWidth=2  IndexOptions=Index vector (dialog)  Indices=[2 1]  OutputSizes=1
  VelocityToOpticalFlow_Gain : Gain  Gain=[0.35 0.35 1]
  opticalFlow_datout : Outport  VectorParamsAs1DForOutWhenUnconnected=off
  wires:
  Demux4/2 -> Product1/1
  Product/1 -> Mux7/1
  Product1/1 -> Mux7/2
  Bus Selector/6 -> Mux8/2  "<VZ>"
  Bus Selector/5 -> Gain2/1  "<Z>"
  Gain1/1 -> Demux4/1
  Demux4/1 -> Product/1
  Gain2/1 -> Product/2, Product1/2
  Mux8/1 -> VelocityToOpticalFlow_Gain/1
  VelocityToOpticalFlow_Gain/1 -> Select dz4/1, Select dz3/1, Select dz2/1
  SwitchPlanarOpticalFlow/1 -> Add1/2
  Add1/1 -> Mux8/1
  Mux2/1 -> Add1/1
  Mux7/1 -> SwitchPlanarOpticalFlow/1
  Select dz2/1 -> Subsystem/1(V_x)
  Select dz3/1 -> Subsystem/3(V_y)
  Subsystem/1(Out1) -> Mux/1
  Subsystem/2(Out2) -> Mux/2
  Mux/1 -> opticalFlow_datout/1
  Select dz4/1 -> Mux/3
  yaw/1 -> Subsystem/2(<yaw>)
  Bus Selector/3 -> Mux1/1  "<p>"
  Bus Selector/4 -> Mux1/2  "<q>"
  Mux1/1 -> Gain1/1
  Bus Selector/1 -> Mux2/1  "<VX>"
  Bus Selector/2 -> Mux2/2  "<VY>"
  pos_att_NED/1 -> Bus Selector/1

== system SiMoDronesBebopRos_student/BEBOP/Measurement block /ROS link + Measure/UDP link/ENU bebop -> NED ==
  <X> : Inport
  <Y> : Inport  Port=2
  <Z> : Inport  Port=3
  Gain : Gain
  Gain1 : Gain
  Gain2 : Gain
  Out1 : Outport  VectorParamsAs1DForOutWhenUnconnected=off
  Out2 : Outport  Port=2  VectorParamsAs1DForOutWhenUnconnected=off
  Out3 : Outport  Port=3  VectorParamsAs1DForOutWhenUnconnected=off
  wires:
  <Z>/1 -> Gain2/1
  <Y>/1 -> Gain1/1
  <X>/1 -> Gain/1
  Gain1/1 -> Out2/1
  Gain/1 -> Out1/1
  Gain2/1 -> Out3/1

== system SiMoDronesBebopRos_student/BEBOP/Model/Model/Acutators1/Motor1 ==
  PWM : Inport
  Bebop drive : lib_isae_drones/Bebop drive  Time_constant=motor.tau_mot  coef_pwm2w=motor.scaling  omega_0=motor.w0  omega_max=motor.wmax
      settings: SourceProductName=ISAE drones
  speed : Outport  VectorParamsAs1DForOutWhenUnconnected=off
  wires:
  Bebop drive/1 -> speed/1
  PWM/1 -> Bebop drive/1

== system SiMoDronesBebopRos_student/BEBOP/Model/Model/Acutators1/Motor2 ==
  PWM : Inport
  Bebop drive : lib_isae_drones/Bebop drive  Time_constant=motor.tau_mot  coef_pwm2w=motor.scaling  omega_0=motor.w0  omega_max=motor.wmax
      settings: SourceProductName=ISAE drones
  speed : Outport  VectorParamsAs1DForOutWhenUnconnected=off
  wires:
  PWM/1 -> Bebop drive/1
  Bebop drive/1 -> speed/1

== system SiMoDronesBebopRos_student/BEBOP/Model/Model/Acutators1/Motor3 ==
  PWM : Inport
  Bebop drive : lib_isae_drones/Bebop drive  Time_constant=motor.tau_mot  coef_pwm2w=motor.scaling  omega_0=motor.w0  omega_max=motor.wmax
      settings: SourceProductName=ISAE drones
  speed : Outport  VectorParamsAs1DForOutWhenUnconnected=off
  wires:
  Bebop drive/1 -> speed/1
  PWM/1 -> Bebop drive/1

== system SiMoDronesBebopRos_student/BEBOP/Model/Model/Acutators1/Motor4 ==
  PWM : Inport
  Bebop drive : lib_isae_drones/Bebop drive  Time_constant=motor.tau_mot  coef_pwm2w=motor.scaling  omega_0=motor.w0  omega_max=motor.wmax
      settings: SourceProductName=ISAE drones
  speed : Outport  VectorParamsAs1DForOutWhenUnconnected=off
  wires:
  PWM/1 -> Bebop drive/1
  Bebop drive/1 -> speed/1

== system SiMoDronesBebopRos_student/OPTITRACK/ROS link + Measure/UDP link/optitrack_pos_vel_uav/Computes velocities ==
  pos_OT : Inport
  computes_vel : MATLAB Function  TreatAsAtomicUnit=on
  vel_OT : Outport  VectorParamsAs1DForOutWhenUnconnected=off
  wires:
  pos_OT/1 -> computes_vel/1(pos_OT)
  computes_vel/1(vel_OT) -> vel_OT/1

== system SiMoDronesBebopRos_student/BEBOP/Bebop Control/Inner Loop (Parrot)/Bebop onboard control/Régulations/Attitude ==
  note: ATTITUDE
  refAttitude : Inport
  att_estim : Inport  Port=2
  rate : Inport  Port=3
  Add : Sum  Inputs=+-
  D_pr : Gain  Gain=[thetaKD;phiKD]
  Delay : Delay  DelayLength=1  InitialCondition=0
  Demux : Demux  Outputs=2
  Discrete-Time Integrator : DiscreteIntegrator  SampleTime=Ts_bebop  LimitOutput=on  UpperSaturationLimit=2  LowerSaturationLimit=-2  ICPrevOutput=DiscIntNeverNeededParam  ICPrevScaledInput=DiscIntNeverNeededParam
  Gain : Gain  Gain=0.8
  P_pr : Gain  Gain=[thetaKP;phiKP]
  P_pr1 : Gain  Gain=[thetaKI;phiKI]
  Scope2 : Scope  NumInputPorts=2
  Sum16 : Sum  Inputs=++-  OutDataTypeStr=Inherit: Inherit via back propagation  SaturateOnIntegerOverflow=on
  Sum19 : Sum  Inputs=+-|
  antiWU_Gain : Gain  Gain=0.001
  tau_pitch : Outport  VectorParamsAs1DForOutWhenUnconnected=off
  tau_roll : Outport  Port=2  VectorParamsAs1DForOutWhenUnconnected=off
  wires:
  Sum16/1 -> Demux/1  "P_pr"
  antiWU_Gain/1 -> Add/2
  Add/1 -> Discrete-Time Integrator/1
  P_pr/1 -> Sum16/1
  P_pr1/1 -> Sum16/2
  Sum19/1 -> Add/1, P_pr/1  "pitch/roll error"
  Discrete-Time Integrator/1 -> Delay/1, P_pr1/1
  Delay/1 -> antiWU_Gain/1
  Demux/1 -> Scope2/1, tau_pitch/1  "tau_pitch"
  Demux/2 -> tau_roll/1, Scope2/2
  D_pr/1 -> Sum16/3
  refAttitude/1 -> Sum19/1
  att_estim/1 -> Sum19/2
  rate/1 -> Gain/1
  Gain/1 -> D_pr/1

== system SiMoDronesBebopRos_student/BEBOP/Bebop Control/Inner Loop (Parrot)/Bebop onboard control/Vz control/Altitude control ==
  note: ATTITUDE
  Vz_ref : Inport
  Motor_On : Inport  Port=2
  Vz_est : Inport  Port=3
  Add : Sum  Inputs=+-
  Delay : Delay  DelayLength=1  InitialCondition=0
  Discrete-Time Integrator : DiscreteIntegrator  ExternalReset=rising  SampleTime=Ts_bebop  LimitOutput=on  UpperSaturationLimit=2  LowerSaturationLimit=-2  ICPrevOutput=DiscIntNeverNeededParam  ICPrevScaledInput=DiscIntNeverNeededParam
  Motor_On1 : InportShadow  Port=2
  P_pr : Gain  Gain=altiKP
  P_pr1 : Gain  Gain=altiKI
  Product : Product
  Sum16 : Sum  Inputs=++|  AccumDataTypeStr=single  OutDataTypeStr=single  SaturateOnIntegerOverflow=on
  Sum19 : Sum  Inputs=+-|
  antiWU_Gain : Gain  Gain=0.001
  Vertical thrust (N) : Outport  VectorParamsAs1DForOutWhenUnconnected=off
  wires:
  antiWU_Gain/1 -> Add/2
  Add/1 -> Discrete-Time Integrator/1
  P_pr/1 -> Sum16/1
  P_pr1/1 -> Sum16/2
  Sum19/1 -> Add/1, P_pr/1  "Vz error"
  Discrete-Time Integrator/1 -> Delay/1, P_pr1/1
  Delay/1 -> antiWU_Gain/1
  Sum16/1 -> Product/1
  Vz_ref/1 -> Sum19/1
  Vz_est/1 -> Sum19/2
  Motor_On/1 -> Discrete-Time Integrator/2
  Motor_On1/1 -> Product/2
  Product/1 -> Vertical thrust (N)/1

== system SiMoDronesBebopRos_student/BEBOP/Bebop Control/Inner Loop (Parrot)/Bebop onboard control/Vz control/Normalized thrust calculation ==
  Vertical thrust : Inport
  theta : Inport  Port=2
  phi : Inport  Port=3
  Constant : Constant  Value=aero.g
  Constant2 : Constant  Value=drone.mtot/4
  Gain : Gain  Gain=1/motor.Pw
  Gain2 : Gain  Gain=-1
  Gain5 : Gain  Gain=1/motor.scaling
  MATLAB Function : MATLAB Function  TreatAsAtomicUnit=on  SystemSampleTime=Ts_bebop
  Product : Product
  Saturation2 : Saturate  UpperLimit=0.7  LowerLimit=0.35
  Saturation3 : Saturate  UpperLimit=1000*1000  LowerLimit=200*200
  Sqrt1 : Sqrt  SaturateOnIntegerOverflow=on
  Sum : Sum  Inputs=|+-
  Normalized thrust : Outport  SampleTime=Ts_bebop  VectorParamsAs1DForOutWhenUnconnected=off
  wires:
  MATLAB Function/1(y) -> Gain/1
  Constant/1 -> Sum/2
  Vertical thrust/1 -> Sum/1
  Gain2/1 -> Product/2
  Sum/1 -> Gain2/1
  Product/1 -> MATLAB Function/1(F)  "F_mot"
  Sqrt1/1 -> Gain5/1
  Saturation2/1 -> Normalized thrust/1
  Gain5/1 -> Saturation2/1
  Saturation3/1 -> Sqrt1/1
  Gain/1 -> Saturation3/1
  Constant2/1 -> Product/1
  theta/1 -> MATLAB Function/2(theta)
  phi/1 -> MATLAB Function/3(phi)

== system SiMoDronesBebopRos_student/BEBOP/Bebop Control/Inner Loop (Parrot)/Bebop onboard control/Vz control/Subsystem ==
  Vz_ref : Inport
  bebop_state : Inport  Port=2
  altitude : Inport  Port=3
  MATLAB Function1 : MATLAB Function  TreatAsAtomicUnit=on
  Rate Transition : RateTransition  OutPortSampleTime=Ts_bebop
  Rate Transition1 : RateTransition  OutPortSampleTime=Ts_bebop
  Vz_ref_out : Outport  VectorParamsAs1DForOutWhenUnconnected=off
  Motor_On : Outport  Port=2  VectorParamsAs1DForOutWhenUnconnected=off
  wires:
  Vz_ref/1 -> MATLAB Function1/1(Vz_ref_in)
  bebop_state/1 -> MATLAB Function1/2(bebop_state)
  MATLAB Function1/1(Vz_ref_out) -> Rate Transition/1  "vz_ref_out"
  MATLAB Function1/2(Motor_on) -> Rate Transition1/1  "Motor_on"
  Rate Transition/1 -> Vz_ref_out/1
  Rate Transition1/1 -> Motor_On/1
  altitude/1 -> MATLAB Function1/3(altitude)

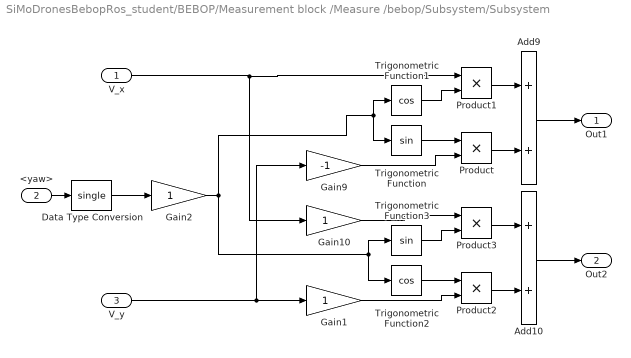
== system SiMoDronesBebopRos_student/BEBOP/Measurement block /Measure /bebop/Subsystem/Subsystem ==
  V_x : Inport
  <yaw> : Inport  Port=2
  V_y : Inport  Port=3
  Add10 : Sum
  Add9 : Sum
  Data Type Conversion : DataTypeConversion  OutDataTypeStr=single
  Gain1 : Gain
  Gain10 : Gain
  Gain2 : Gain
  Gain9 : Gain  Gain=-1
  Product{,1..3} (4 alike) : Product
  Trigonometric Function : Trigonometry
  Trigonometric Function1 : Trigonometry  Operator=cos
  Trigonometric Function2 : Trigonometry  Operator=cos
  Trigonometric Function3 : Trigonometry
  Out1 : Outport  VectorParamsAs1DForOutWhenUnconnected=off
  Out2 : Outport  Port=2  VectorParamsAs1DForOutWhenUnconnected=off
  wires:
  Gain2/1 -> Trigonometric Function/1, Trigonometric Function1/1, Trigonometric Function2/1, Trigonometric Function3/1
  V_x/1 -> Product1/1, Gain10/1
  V_y/1 -> Gain9/1, Gain1/1
  Add9/1 -> Out1/1
  Product/1 -> Add9/2
  Product1/1 -> Add9/1
  Trigonometric Function/1 -> Product/1
  Trigonometric Function1/1 -> Product1/2
  Add10/1 -> Out2/1
  Product2/1 -> Add10/2
  Product3/1 -> Add10/1
  Trigonometric Function2/1 -> Product2/1
  Trigonometric Function3/1 -> Product3/2
  Gain9/1 -> Product/2
  Gain10/1 -> Product3/1
  <yaw>/1 -> Data Type Conversion/1
  Gain1/1 -> Product2/2
  Data Type Conversion/1 -> Gain2/1

== matlab function SiMoDronesBebopRos_student/BEBOP/Bebop Control/Inner Loop (Parrot)/Bebop onboard control/Vz control/Normalized thrust calculation/MATLAB Function ==
  data: F input; y output; theta input; phi input
function y = fcn(F,theta,phi)

y = F/(cos(theta)*cos(phi));

== matlab function SiMoDronesBebopRos_student/BEBOP/Bebop Control/Udp send/Topics/MATLAB Function ==
  data: e1 input; TAKE_OFF output; e2 input; LAND output
function [TAKE_OFF, LAND] = fcn(e1,e2)

s1=e1;
s2=e2;

if e1==e2
    e1=0;
end

    
TAKE_OFF=e1;
LAND=e2;

== matlab function SiMoDronesBebopRos_student/BEBOP/Measurement block /Measure /bebop/MATLAB Function1 ==
  data: in input; out output
function out = fcn(in)
%#codegen

%y = mod(u+pi, 2*pi) - pi;

if (in < -pi) || (pi < in)
    out = in + pi;
    out = mod(out, 2*pi) - pi;
else
    out = in;
end
